simulink model "CBB_ccontrol_pspice_PI_NOLINEAL"  (R2021a)
settings: Solver=VariableStepAuto  StartTime=0.0  StopTime=1  RelTol=1e-3
undefined symbols (not defined in the file): delta1, delta2, id, kp, L, R
libraries: pspsim x1, spsSawtoothGeneratorLib x1
settings Model: Creator=Omar_Chavez  LastModifiedBy=omar_

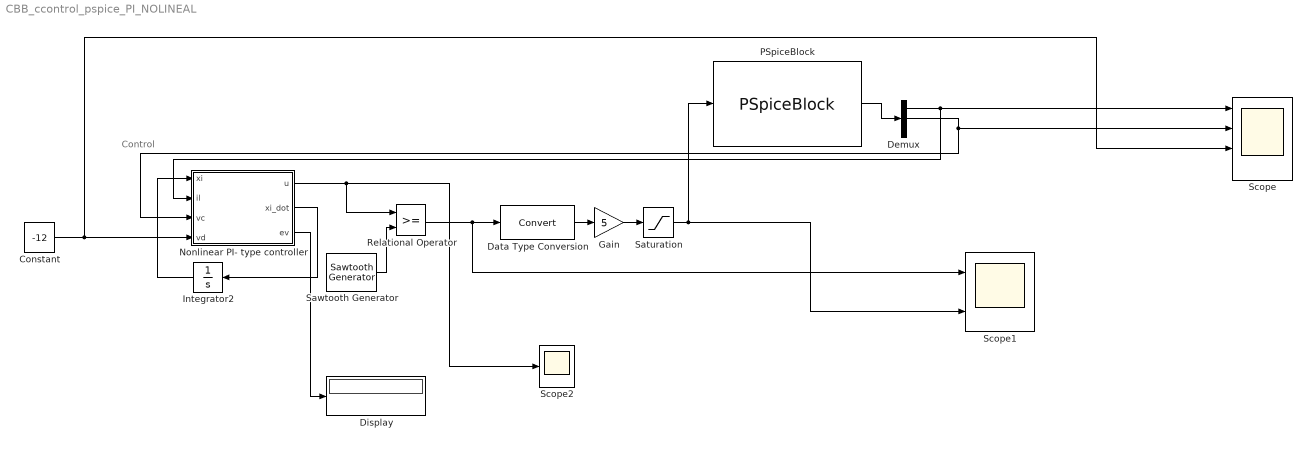
== system CBB_ccontrol_pspice_PI_NOLINEAL ==
  note: Control
  Constant : Constant  Value=-12
  Data Type Conversion : DataTypeConversion
  Demux : Demux  Outputs=3
  Display : Display
  Gain : Gain  Gain=5
  Integrator2 : Integrator  InitialCondition=0.001
  "Nonlinear PI- type controller " : MATLAB Function  TreatAsAtomicUnit=on
  PSpiceBlock : pspsim/PSpiceBlock  SFunctionModules=''
      settings: SourceProductName=PSpice Block
  Relational Operator : RelationalOperator  OutDataTypeStr=boolean  RndMeth=Simplest
  Saturation : Saturate  UpperLimit=5  LowerLimit=0
  Sawtooth Generator : spsSawtoothGeneratorLib/Sawtooth Generator  Freq=50000  Phase=0  Ts=0
  Scope : Scope  NumInputPorts=4
  Scope1 : Scope  NumInputPorts=2
  Scope2 : Scope  NumInputPorts=3
  wires:
  Constant/1 -> Scope/3, "Nonlinear PI- type controller "/4(vd)
  "Nonlinear PI- type controller "/1(u) -> Relational Operator/1, Scope2/2
  "Nonlinear PI- type controller "/2(xi_dot) -> Integrator2/1
  Sawtooth Generator/1 -> Relational Operator/2
  Integrator2/1 -> "Nonlinear PI- type controller "/1(xi)
  PSpiceBlock/1 -> Demux/1
  Demux/1 -> Scope/1, "Nonlinear PI- type controller "/2(il)
  Demux/2 -> Scope/2, "Nonlinear PI- type controller "/3(vc)
  Data Type Conversion/1 -> Gain/1
  Relational Operator/1 -> Scope1/1, Data Type Conversion/1
  Gain/1 -> Saturation/1
  Saturation/1 -> Scope1/2, PSpiceBlock/1
  "Nonlinear PI- type controller "/3(ev) -> Display/1

== matlab function CBB_ccontrol_pspice_PI_NOLINEAL/Nonlinear PI- type controller  ==
  data: E parameter; u output; xi_dot output; delta2 parameter; R parameter; kp parameter; delta1 parameter; id parameter; xi input; il input; vc input; L parameter; vd input; ev output
function [u,xi_dot,ev] = fcn(E, delta2, R, kp, delta1, id, xi,il,vc,L, vd)

il = double(il); vc = double(vc);
ei_s = double(il - id - xi); ev = double(vc -vd);


gamma  = (delta1 - delta2)/(L*delta1*delta2);
phi = -kp*((delta1*(E - vd)*ei_s) + delta2*vd*((vd-E)/R*E)*ev );
xi_dot = -gamma*delta2*((E/(vd - E)+ phi)*ev);
u = (vd/(vd-E))+ phi;
